simulink library "roombaLibrary"  (R2017b)
settings: Solver=VariableStepAuto  StartTime=0.0  StopTime=10.0  RelTol=1e-3
settings Model: Creator=ibrahim  LastModifiedBy=wafflefries
settings CodeAppCC: StateflowObjectComments=on

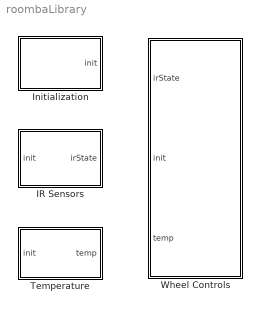
== system roombaLibrary ==
  "IR Sensors " : Subsystem
  Initialization : Subsystem
  Temperature : Subsystem
  Wheel Controls : Subsystem

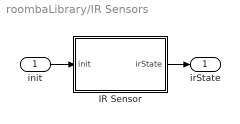
== system roombaLibrary/IR Sensors  ==
  init : Inport
  IR Sensor : Stateflow chart  TreatAsAtomicUnit=on
  irState : Outport
  wires:
  IR Sensor/1(irState) -> irState/1
  init/1 -> IR Sensor/1(init)

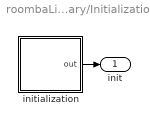
== system roombaLibrary/Initialization ==
  initialization : Stateflow chart  AncestorBlock=untitled/Init/Chart  TreatAsAtomicUnit=on
  init : Outport
  wires:
  initialization/1(out) -> init/1

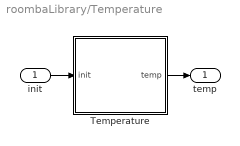
== system roombaLibrary/Temperature ==
  init : Inport
  Temperature : Stateflow chart  TreatAsAtomicUnit=on
  temp : Outport
  wires:
  init/1 -> Temperature/1(init)
  Temperature/1(temp) -> temp/1

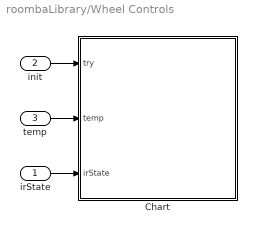
== system roombaLibrary/Wheel Controls ==
  irState : Inport
  init : Inport  Port=2
  temp : Inport  Port=3
  Chart : Stateflow chart  TreatAsAtomicUnit=on
  wires:
  init/1 -> Chart/1(try)
  temp/1 -> Chart/2(temp)
  irState/1 -> Chart/3(irState)

== stateflow chart roombaLibrary/Temperature/Temperature ==
  state temp
    en,du:
    temp=T;
  (default) -> temp
  data: y function_output; init input; temp output
  function y=T:
    | function y=T
    | y=0;
    | persistent obj
    | coder.extrinsic('evalin');
    | coder.extrinsic('get');
    | if isempty(obj)
    |     obj = evalin('base','objWs');
    | end
    | coder.extrinsic('TemperatureRoomba');
    | y=TemperatureRoomba(obj);

== stateflow chart roombaLibrary/IR Sensors /IR Sensor ==
  state SCAN
    en,du:
    irState=IR;
  (default) -> SCAN
  data: y function_output; init input double; irState output
  function y=IR:
    | function y=IR
    | y=[0,0,0,0,0,0];
    | persistent obj
    | coder.extrinsic('evalin');
    | coder.extrinsic('get');
    | if isempty(obj)
    |     obj = evalin('base','objWs');
    | end
    | coder.extrinsic('RangeStateRoomba');
    | y=RangeStateRoomba(obj);

== stateflow chart roombaLibrary/Initialization/initialization ==
  state START
    en,du:
    tcpInit;
    out=1;
  (default) -> START
  data: out output
  function tcpInit:
    | function tcpInit
    | coder.extrinsic('RoombaWiFiInit');
    | coder.extrinsic('assignin');
    | persistent obj
    | if isempty(obj)
    |     obj=RoombaWiFiInit('10.0.0.1','full');
    |     assignin('base','objWs',obj);
    | end

== stateflow chart roombaLibrary/Wheel Controls/Chart ==
  state START
    state OFF
      en,du:
      Wheels(0,0);
    state ON
      state REV
        entry:
        Wheels(-0.1,-0.1);
      state FWD
        entry,du:
        Wheels(0.04,0.04);
      state R2
        entry,du:
        Wheels(-0.2,0.3);
      state R1
        entry,du:
        Wheels(-0.1,0.2);
      state R3
        entry,du:
        Wheels(-0.2,0.2);
      state L3
        entry,du:
        Wheels(0.2,-0.2);
      state L2
        entry,du:
        Wheels(0.3,-0.2);
      state L1
        entry,du:
        Wheels(0.2,-0.1);
      (default) -> REV
      REV -> FWD : after(1,sec)
      FWD -> R1 [order 1] : [irState(1)>0]
      R1 -> FWD : [irState(1)<1]
      FWD -> R2 [order 2] : [irState(2)>0]
      R2 -> FWD : [irState(2)<1]
      FWD -> R3 [order 3] : [irState(3)>0]
      R3 -> FWD : [irState(3)<1]
      FWD -> L3 [order 4] : [irState(4)>0]
      L3 -> FWD : [irState(4)<1]
      FWD -> L2 [order 5] : [irState(5)>0]
      L2 -> FWD : [irState(5)<1]
      FWD -> L1 [order 6] : [irState(6)>0]
      L1 -> FWD : [irState(6)<1]
    (default) -> OFF
    OFF -> ON : [temp<75]
    ON -> OFF : [temp>=75]
  (default) -> START
  data: u1 function_input; u2 function_input; try input; temp input; irState input
  function Wheels(u1,u2):
    | function Wheels(u1,u2)
    | persistent so
    | coder.extrinsic('evalin');
    | coder.extrinsic('get');
    | so = evalin('base','objWs');
    | coder.extrinsic('SetWheelVelRoomba');
    | SetWheelVelRoomba(so,u1,u2);
